simulink model "new_nncontroller_5_30"  (R2021a)
settings: Solver=VariableStepAuto  StartTime=0.0  StopTime=10.0  RelTol=1e-3
libraries: neural x157
(part 10 of 10)

== system new_nncontroller_5_30/Feed-Forward Neural Network/Layer 6/Delays 1 ==
  "p{6}" : Inport  PortDimensions=30
      mask Display: e = 0.06;c1 = [120 230 180]/255;c2 = ([120 230 180]+0)/(256+128);c3 = ([120 230 180]+128)/(256+128);patch([0 1 1 0],[0 0 1 1],c1);patch([0 1 1 1-e 1-e 0+e],[0 0 1 1-e 0+e 0+e],c2);patch([0 0 1 1-e 0+e 0+e],[0 1 1 1-e 1-e 0+e],c3);plot([0 1 1 0 0],[0 0 1 1 0]);
  mux : Mux  Inputs=1
      mask Display: e = 0.06;c1 = [120 150 230]/255;c2 = ([120 150 230]+0)/383;c3 = ([120 150 230]+128)/383;patch([0 1 1 0],[0 0 1 1],c1);patch([0 1 1 1-e 1-e 0+e],[0 0 1 1-e 0+e 0+e],c2);patch([0 0 1 1-e 0+e 0+e],[0 1 1 1-e 1-e 0+e],c3);plot([0 1 1 0 0],[0 0 1 1 0]);disp('Mux')
  "pd{6,5}" : Outport
      mask Display: e = 0.06;c1 = [120 230 180]/255;c2 = ([120 230 180]+0)/(256+128);c3 = ([120 230 180]+128)/(256+128);patch([0 1 1 0],[0 0 1 1],c1);patch([0 1 1 1-e 1-e 0+e],[0 0 1 1-e 0+e 0+e],c2);patch([0 0 1 1-e 0+e 0+e],[0 1 1 1-e 1-e 0+e],c3);plot([0 1 1 0 0],[0 0 1 1 0]);
  wires:
  "p{6}"/1 -> mux/1
  mux/1 -> "pd{6,5}"/1

== system new_nncontroller_5_30/Feed-Forward Neural Network/Layer 6/LW{6,5} ==
  "ad{6,5}" : Inport  PortDimensions=30
      mask Display: e = 0.06;c1 = [120 230 180]/255;c2 = ([120 230 180]+0)/(256+128);c3 = ([120 230 180]+128)/(256+128);patch([0 1 1 0],[0 0 1 1],c1);patch([0 1 1 1-e 1-e 0+e],[0 0 1 1-e 0+e 0+e],c2);patch([0 0 1 1-e 0+e 0+e],[0 1 1 1-e 1-e 0+e],c3);plot([0 1 1 0 0],[0 0 1 1 0]);
  "IW{6,5}(1,:)'" : Constant  Value=[-0.429869884791111100952321066870354115962982177734375;0.68687649610011092260464238279382698237895965576171875;-0.52186564412719860239775471200118772685527801513671875;-0.71589743317965659485935248085297644138336181640625;-0.541367529690830462385520149837248027324676513671875;-0.6858345942777663850620228913612663745880126953125;-0.433998488009012028943089944732491858303546905517578125;-0.09900999703784811589724057512285071425139904022216796875;-0.05527371268078647148502824393290211446583271026611328125;0.4825945995732106030828845177893526852130889892578125;0.375813468591757182668544601256144233047962188720703125;-0.9800176873532944199496341752819716930389404296875;-0.1884688003383645504840160356252454221248626708984375;-0.407575863060370746637772754183970391750335693359375;0.87199027482647506470669895861647091805934906005859375;0.281718039354810656504923827014863491058349609375;-0.417141949459292560309364716886193491518497467041015625;-0.8937773602691432284217398773762397468090057373046875;-0.57737613949521870981840265812934376299381256103515625;-0.1856242035660426170640135978828766383230686187744140625;-0.82063975998461302641118209066917188465595245361328125;0.598891811205529034367600615951232612133026123046875;0.85945526012137618554476148347021080553531646728515625;-0.2363030719355891928756818742840550839900970458984375;0.9942956787278267594132330486900173127651214599609375;-0.59257448017762470726665924303233623504638671875;-0.03735792060762488375758039182983338832855224609375;0.3312520966432785929356441556592471897602081298828125;-0.8776623324084249500032228752388618886470794677734375;-0.3826637676552737676871629446395672857761383056640625]
      mask Display: e = 0.06;c1 = [120 150 230]/255;c2 = ([120 150 230]+0)/383;c3 = ([120 150 230]+128)/383;patch([0 1 1 0],[0 0 1 1],c1);patch([0 1 1 1-e 1-e 0+e],[0 0 1 1-e 0+e 0+e],c2);patch([0 0 1 1-e 0+e 0+e],[0 1 1 1-e 1-e 0+e],c3);plot([0 1 1 0 0],[0 0 1 1 0]);disp('weights');
  Mux : Mux  Inputs=1
      mask Display: e = 0.06;c1 = [120 150 230]/255;c2 = ([120 150 230]+0)/383;c3 = ([120 150 230]+128)/383;patch([0 1 1 0],[0 0 1 1],c1);patch([0 1 1 1-e 1-e 0+e],[0 0 1 1-e 0+e 0+e],c2);patch([0 0 1 1-e 0+e 0+e],[0 1 1 1-e 1-e 0+e],c3);plot([0 1 1 0 0],[0 0 1 1 0]);disp('Mux');
  dotprod1 : neural/Weight Functions/dotprod
  "lz{6,5}" : Outport
      mask Display: e = 0.06;c1 = [120 230 180]/255;c2 = ([120 230 180]+0)/(256+128);c3 = ([120 230 180]+128)/(256+128);patch([0 1 1 0],[0 0 1 1],c1);patch([0 1 1 1-e 1-e 0+e],[0 0 1 1-e 0+e 0+e],c2);patch([0 0 1 1-e 0+e 0+e],[0 1 1 1-e 1-e 0+e],c3);plot([0 1 1 0 0],[0 0 1 1 0]);
  wires:
  "IW{6,5}(1,:)'"/1 -> dotprod1/1
  "ad{6,5}"/1 -> dotprod1/2
  dotprod1/1 -> Mux/1
  Mux/1 -> "lz{6,5}"/1
